simulink model "mig"  (R2021b)
settings: Solver=VariableStepAuto  StartTime=0.0  StopTime=10.0  RelTol=1e-3
undefined symbols (not defined in the file or in its folder): K2_fcem
libraries: spsAsynchronousMachinepuUnitsLib x1
settings Model: Creator=João Gabriel  LastModifiedBy=João Gabriel

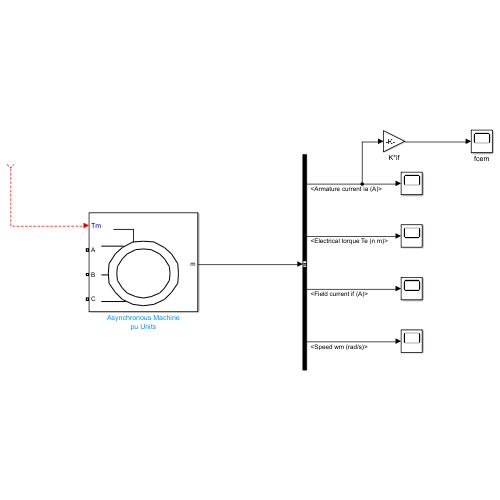
[thumbnail: Simulink's stored preview of the top-level diagram]
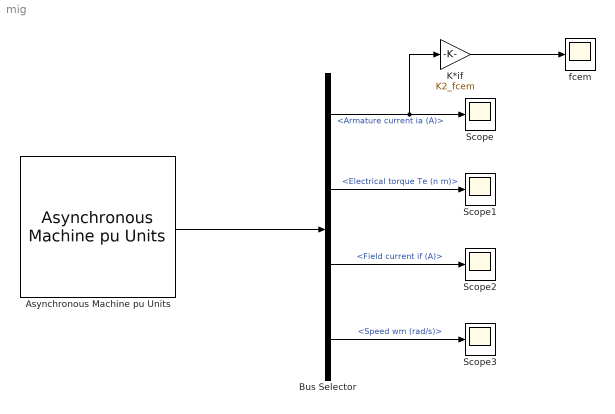
== system mig ==
  Asynchronous Machine pu Units : spsAsynchronousMachinepuUnitsLib/Asynchronous Machine pu Units  RotorType=Squirrel-cage  PresetModel=No  MechanicalLoad=Torque Tm  ShowDetailedParameters=on  ReferenceFrame=Rotor  Units=pu  MeasurementBus=off  NominalParameters=[3730 460 60]  VoltageRatio=1  Stator=[0.01965 0.0397]  Rotor=[0.01909 0.0397]  Cage1=[0.01909 0.0397]  Cage2=[0.01909 0.0397]  Lm=1.354  Mechanical=[0.09526 0.05479 2]  PolePairs=2  InitialConditions="[ 1,0   0,0,0   0,0,0 ]"  SimulateSaturation=off  Saturation="[0.212,0.4201,0.8125,1.0979,1.4799,2.2457,3.2586,4.5763,6.4763 ;   0.5,0.7,0.9,1,1.1,1.2 ,1.3,1.4,1.5]"  LoadFlowParameters=0  TsPowergui=0  TsBlock=-1  IterativeModel=Trapezoidal non iterative  IterativeDiscreteModel=Trapezoidal non iterative  Pmec=0
      settings: SourceProductBaseCode=PS
  Bus Selector : BusSelector  OutputSignals=Armature current ia (A),Electrical torque Te (n m),Field current if (A),Speed wm (rad/s)
  K*if : Gain  Gain=K2_fcem
  Scope{,1..3} (4 alike) : Scope
  fcem : Scope
  wires:
  K*if/1 -> fcem/1
  Bus Selector/3 -> Scope2/1  "<Field current if (A)>"
  Bus Selector/4 -> Scope3/1  "<Speed wm (rad/s)>"
  Bus Selector/1 -> K*if/1, Scope/1  "<Armature current ia (A)>"
  Bus Selector/2 -> Scope1/1  "<Electrical torque Te (n m)>"
  Asynchronous Machine pu Units/1 -> Bus Selector/1
  ? -> Asynchronous Machine pu Units/1
